simulink model "SRR_PD"  (R2024b)
settings: Solver=ode4  StartTime=0.0  StopTime=20.0  FixedStep=0.15  RelTol=1e-3
InitFcn:
  | Kp = 1;
  | Kv = 1;
settings Model: Creator=iamma  LastModifiedBy=iamma

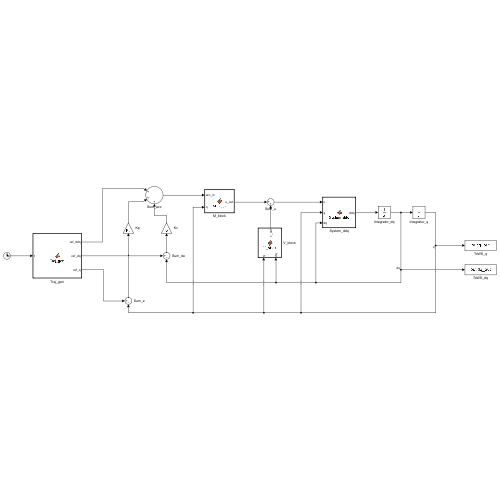
[thumbnail: Simulink's stored preview of the top-level diagram]
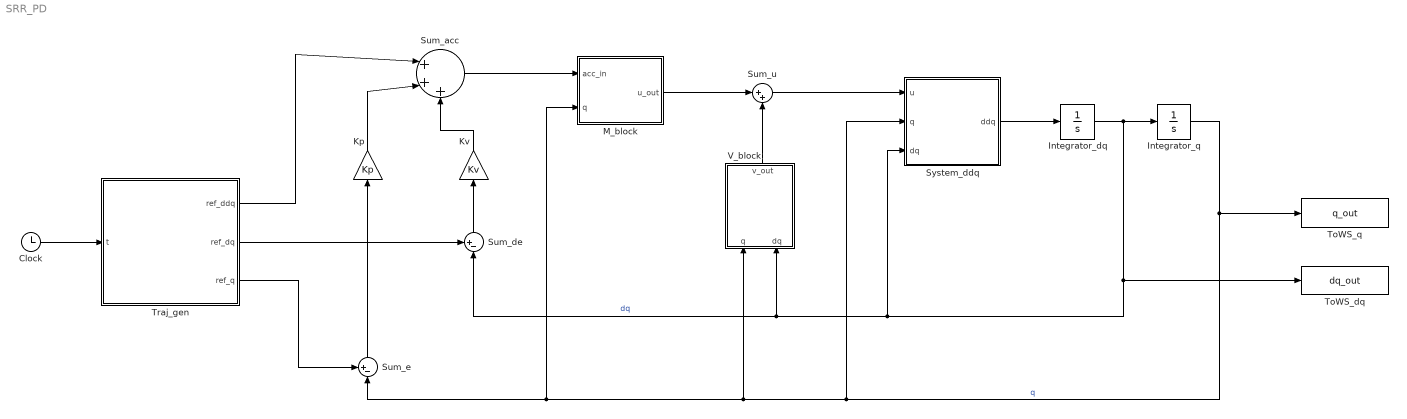
== system SRR_PD ==
  Clock : Clock
  Integrator_dq : Integrator  InitialCondition=zeros(4, 1)
  Integrator_q : Integrator  InitialCondition=zeros(4, 1)
  Kp : Gain  Gain=Kp
  Kv : Gain  Gain=Kv
  M_block : MATLAB Function  TreatAsAtomicUnit=on
  Sum_acc : Sum  Inputs=||+|+|+
  Sum_de : Sum  Inputs=+-|
  Sum_e : Sum  Inputs=+-|
  Sum_u : Sum  Inputs=|++
  System_ddq : MATLAB Function  TreatAsAtomicUnit=on
  ToWS_dq : ToWorkspace  VariableName=dq_out  SampleTime=-1
      settings: Save2DSignal=2-D array (concatenate along first dimension)
  ToWS_q : ToWorkspace  VariableName=q_out  SampleTime=-1
      settings: Save2DSignal=2-D array (concatenate along first dimension)
  Traj_gen : MATLAB Function  TreatAsAtomicUnit=on
  V_block : MATLAB Function  TreatAsAtomicUnit=on
  wires:
  Traj_gen/1(ref_ddq) -> Sum_acc/1
  Traj_gen/2(ref_dq) -> Sum_de/1
  Sum_de/1 -> Kv/1
  Kv/1 -> Sum_acc/3
  Traj_gen/3(ref_q) -> Sum_e/1
  Sum_e/1 -> Kp/1
  Kp/1 -> Sum_acc/2
  Sum_acc/1 -> M_block/1(acc_in)
  M_block/1(u_out) -> Sum_u/1
  V_block/1(v_out) -> Sum_u/2
  Sum_u/1 -> System_ddq/1(u)
  System_ddq/1(ddq) -> Integrator_dq/1
  Integrator_dq/1 -> ToWS_dq/1, System_ddq/3(dq), V_block/2(dq), Sum_de/2, Integrator_q/1  "dq"
  Integrator_q/1 -> ToWS_q/1, V_block/1(q), M_block/2(q), Sum_e/2, System_ddq/2(q)  "q"
  Clock/1 -> Traj_gen/1(t)

== matlab function SRR_PD/M_block ==
  data: acc_in input; u_out output; q input
function u_out = M_block(acc_in, q)
% M(q) * acc_in
p = get_params();
M = calc_M(q, p);
u_out = M * acc_in;
end

== matlab function SRR_PD/System_ddq ==
  data: u input; ddq output; q input; dq input
function ddq = System_ddq(u, q, dq)
% ddq = M^{-1} * (u - V)
p = get_params();
M = calc_M(q, p);
V = calc_V(q, dq, p);
ddq = M \ (u - V);
end

== matlab function SRR_PD/Traj_gen ==
  data: t input; ref_ddq output; ref_dq output; ref_q output
function [ref_ddq, ref_dq, ref_q] = Traj_gen(t)
[ref_ddq, ref_dq, ref_q] = traj_circular(t);
end

== matlab function SRR_PD/V_block ==
  data: q input; dq input; v_out output
function v_out = V_block(q, dq)
% V(q, dq) 비선형 항
p = get_params();
v_out = calc_V(q, dq, p);
end
